simulink model "PIDdesign"  (R2019b)
settings: Solver=VariableStepAuto  StartTime=0.0  StopTime=5  RelTol=1e-3
values from neighbouring files (symbols this model uses):
  F2 = a*mass*g/(a+b)    (= 14.8072837402)    [main.m]
  g = 9.8    [EOM.m]    (also in main.m = 9.81)
  KDX = DesignVars(1,1).Value    [pidOptimization.m]
  KDY = DesignVars(2,1).Value    [pidOptimization.m]
  KIX = DesignVars(3,1).Value    [pidOptimization.m]
  KIY = DesignVars(4,1).Value    [pidOptimization.m]
  Kps = (Vmax-Vmin)/(Hmax-Hmin)    (= 1666.66666667)    [main.m]
  KPX = DesignVars(5,1).Value    [pidOptimization.m]
  KPY = DesignVars(6,1).Value    [pidOptimization.m]
  Ksv = 30    [main.m]
  nu = 1/h0    (= 20000)    [main.m]
  tau = 0.12    [main.m]
  Ts = 1/fs    (= 0.001)    [main.m]
  xeq = x(end,1)    [main.m]
  yeq = x(end,3)    [main.m]
undefined symbols (not defined in the file or in its folder): DiscIntNeverNeededParam
libraries: neural x106, simulink x4, checkpacklib x2
(part 3 of 3)

== system PIDdesign/NONLINEAR BEARING #2 WITHOUT UNBALANCE/BEARING 2 NL/B2NN/Layer 2/Delays 1 ==
  "p{2}" : Inport  PortDimensions=100
      mask Display: e = 0.06;c1 = [120 230 180]/255;c2 = ([120 230 180]+0)/(256+128);c3 = ([120 230 180]+128)/(256+128);patch([0 1 1 0],[0 0 1 1],c1);patch([0 1 1 1-e 1-e 0+e],[0 0 1 1-e 0+e 0+e],c2);patch([0 0 1 1-e 0+e 0+e],[0 1 1 1-e 1-e 0+e],c3);plot([0 1 1 0 0],[0 0 1 1 0]);
  mux : Mux  Inputs=1
      mask Display: e = 0.06;c1 = [120 150 230]/255;c2 = ([120 150 230]+0)/383;c3 = ([120 150 230]+128)/383;patch([0 1 1 0],[0 0 1 1],c1);patch([0 1 1 1-e 1-e 0+e],[0 0 1 1-e 0+e 0+e],c2);patch([0 0 1 1-e 0+e 0+e],[0 1 1 1-e 1-e 0+e],c3);plot([0 1 1 0 0],[0 0 1 1 0]);disp('Mux')
  "pd{2,1}" : Outport
      mask Display: e = 0.06;c1 = [120 230 180]/255;c2 = ([120 230 180]+0)/(256+128);c3 = ([120 230 180]+128)/(256+128);patch([0 1 1 0],[0 0 1 1],c1);patch([0 1 1 1-e 1-e 0+e],[0 0 1 1-e 0+e 0+e],c2);patch([0 0 1 1-e 0+e 0+e],[0 1 1 1-e 1-e 0+e],c3);plot([0 1 1 0 0],[0 0 1 1 0]);
  wires:
  "p{2}"/1 -> mux/1
  mux/1 -> "pd{2,1}"/1

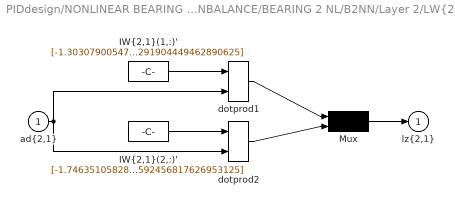
== system PIDdesign/NONLINEAR BEARING #2 WITHOUT UNBALANCE/BEARING 2 NL/B2NN/Layer 2/LW{2,1} ==
  "ad{2,1}" : Inport  PortDimensions=100
      mask Display: e = 0.06;c1 = [120 230 180]/255;c2 = ([120 230 180]+0)/(256+128);c3 = ([120 230 180]+128)/(256+128);patch([0 1 1 0],[0 0 1 1],c1);patch([0 1 1 1-e 1-e 0+e],[0 0 1 1-e 0+e 0+e],c2);patch([0 0 1 1-e 0+e 0+e],[0 1 1 1-e 1-e 0+e],c3);plot([0 1 1 0 0],[0 0 1 1 0]);
  "IW{2,1}(1,:)'" : Constant  Value=[-1.303079005476538210217540836310945451259613037109375;-0.8255005328617783799671769884298555552959442138671875;2.2416068989862178995053909602575004100799560546875;-0.55813390794967288055516974054626189172267913818359375;1.7083747820462615862879829364828765392303466796875;-5.33271180681637968490349521744064986705780029296875;1.93314459538238825331291081965900957584381103515625;-4.29747102149679438554130683769471943378448486328125;-1.835974747092809167270388570614159107208251953125;1.6115522585205634964466980818542651832103729248046875;-0.96088665944156925746710840030573308467864990234375;3.081953249444248310595639850362204015254974365234375;0.40542445031319385151391543331556022167205810546875;-2.371372573954384055383570739650167524814605712890625;0.2222251558369831292427676316947326995432376861572265625;-3.2786957332744872672947167302481830120086669921875;-0.65721019194913754546405471046455204486846923828125;4.5793081924106235902627304312773048877716064453125;3.396559076337279936552704384666867554187774658203125;-0.9506936842022923883632756769657135009765625;0.035530059029697712291717692778547643683850765228271484375;3.669635786509892749762684616143815219402313232421875;-1.0406028671959399733992768233292736113071441650390625;6.63327812826948548519112591748125851154327392578125;3.2833077579783580546290977508760988712310791015625;-1.003788449281528993850542974541895091533660888671875;1.5295131093832996516113098550704307854175567626953125;-0.292529913673766850390478566623642109334468841552734375;0.0103447720973679491152097398298792541027069091796875;-2.094937264749708649702597540454007685184478759765625;2.884830698716304819839706397033296525478363037109375;3.610348251303457711713917888118885457515716552734375;-0.65402756814988738387484090708312578499317169189453125;-0.2477855440938181164067799500116962008178234100341796875;1.469517455897823676735924891545437276363372802734375;-4.46176275310569980803165890392847359180450439453125;3.424182043452276946737811158527620136737823486328125;-5.45843716066573581002785431337542831897735595703125;-6.33904303768679344699421562836505472660064697265625;-4.5012635128892153346669147140346467494964599609375;3.136120918716373662249452536343596875667572021484375;1.571961496786693057714501264854334294795989990234375;-0.23371558494610022993498432697379030287265777587890625;-0.4635484960930360553987839011824689805507659912109375;3.23848369610364361648180420161224901676177978515625;2.509785332547937120040160152711905539035797119140625;2.960969019394504631037534636561758816242218017578125;3.81271075753365362714930597576312720775604248046875;0.87046392166746577867542100648279301822185516357421875;2.527528429159737743958658029441721737384796142578125;2.334886902139819309098811572766862809658050537109375;-2.2202064604060733898904800298623740673065185546875;-1.0971350826732237937477520972606725990772247314453125;5.3252075174508259891581474221311509609222412109375;1.9927529899432936399961135975900106132030487060546875;-1.7323109900493751656114227444049902260303497314453125;-5.2127254975364589739683651714585721492767333984375;3.613077625658748903703099131234921514987945556640625;-2.971965610222664366801836877129971981048583984375;1.9566041764405515124281009775586426258087158203125;0.8251166177697630832454933624831028282642364501953125;0.1193121441991285835992897546020685695111751556396484375;4.02380804450181717157875027623958885669708251953125;-1.0438645216073492161257263433071784675121307373046875;-0.477159922080958420753660220725578255951404571533203125;0.37484864586592514523744057441945187747478485107421875;-2.07618859433052183049994710017926990985870361328125;-3.19484410683969688449224122450686991214752197265625;0.5047112998937421934897429309785366058349609375;-0.181158393879384760349893213060568086802959442138671875;-3.09578760470798641790679539553821086883544921875;-1.4108370343958658299499120403197593986988067626953125;0.146634116610219356058308903811848722398281097412109375 ...(+1495 chars)]
      mask Display: e = 0.06;c1 = [120 150 230]/255;c2 = ([120 150 230]+0)/383;c3 = ([120 150 230]+128)/383;patch([0 1 1 0],[0 0 1 1],c1);patch([0 1 1 1-e 1-e 0+e],[0 0 1 1-e 0+e 0+e],c2);patch([0 0 1 1-e 0+e 0+e],[0 1 1 1-e 1-e 0+e],c3);plot([0 1 1 0 0],[0 0 1 1 0]);disp('weights');
  "IW{2,1}(2,:)'" : Constant  Value=[-1.7463510582880579224962502848939038813114166259765625;-0.3817553257546679734701911002048291265964508056640625;1.499441293389509155531413853168487548828125;0.59781227902492417580759820339153520762920379638671875;-1.572959088991725540296329199918545782566070556640625;-2.285896302660940904161179787479341030120849609375;0.1226153749453533225999279920870321802794933319091796875;0.48879224355486050601626857314840890467166900634765625;1.78087930741924349575810992973856627941131591796875;4.90264426696804722638489693053998053073883056640625;0.1678230741406869508391963563553872518241405487060546875;-5.99359077138990858912848125328309834003448486328125;-0.209639533671976519002555505721829831600189208984375;-0.8073258432726018174463433751952834427356719970703125;5.99096088644159152636348153464496135711669921875;1.47211352452196830853381470660679042339324951171875;4.13072350460404269512082464643754065036773681640625;1.3951298877763722572353799478150904178619384765625;0.267840609452006772617238539169193245470523834228515625;0.514410507555337570551046155742369592189788818359375;-8.597222996447595022573295864276587963104248046875;0.307005832961274205405999282447737641632556915283203125;1.0845127341180493818484364965115673840045928955078125;0.310722374666608847082471811518189497292041778564453125;1.1956344181233660162178011887590400874614715576171875;5.717061542137354734904874931089580059051513671875;-0.7872353439733881241835433684173040091991424560546875;-0.061544718284544497333143908690544776618480682373046875;-1.9906366295749784445234809027169831097126007080078125;-1.22258124482643903974121712963096797466278076171875;-1.515291638847875876905391123727895319461822509765625;2.7375042395839752629171925946138799190521240234375;-2.12826270114527460464159958064556121826171875;3.76220142421134529087112241541035473346710205078125;1.19249507911392971237773963366635143756866455078125;7.46450533719423159340067286393605172634124755859375;-1.57667617645866275921662236214615404605865478515625;0.13616106452400511539480021383496932685375213623046875;-0.03129722684529256948593456399976275861263275146484375;3.924354752442267280088117331615649163722991943359375;-6.7691416449166137425663691828958690166473388671875;1.455619350448965843014548227074556052684783935546875;0.1525039889476383636601752868955372832715511322021484375;3.81711921888099414701400746707804501056671142578125;-3.98679521713969808871524946880526840686798095703125;-4.23988796601051287638028952642343938350677490234375;1.1313598364804284823748048438574187457561492919921875;1.1338509882875762446730050214682705700397491455078125;-1.2873351419050964583590257461764849722385406494140625;-9.5250529974971502866765149519778788089752197265625;0.5386492857873672601698444850626401603221893310546875;-2.911503092256425784256634869961999356746673583984375;0.2278597588163693010709920372391934506595134735107421875;1.127643531196385051629249574034474790096282958984375;0.55780526308049738215544266495271585881710052490234375;5.93775110923110371885513814049772918224334716796875;0.16441798355035242007460283275577239692211151123046875;2.51670428144922642132996770669706165790557861328125;3.690456488905490051166680132155306637287139892578125;-6.58276106105876124274800531566143035888671875;-2.462614925171888291544064486515708267688751220703125;5.5107188605968957517688977532088756561279296875;1.381019801933926149928311133407987654209136962890625;4.75763931600114187148165001417510211467742919921875;-2.782763876646672684955774457193911075592041015625;3.306763994148273599904541697469539940357208251953125;-0.186539850676508522919760935110389254987239837646484375;3.029849029120091241651380187249742448329925537109375;0.2916556119648117118003938230685889720916748046875;1.9746781314328030187965623554191552102565765380859375;-1.8717633335384376014332019622088409960269927978515625;1.3419353608102879693575459896237589418888092041015625;-0.74501009632939396709616630687378346920013427734375 ...(+1460 chars)]
      mask Display: e = 0.06;c1 = [120 150 230]/255;c2 = ([120 150 230]+0)/383;c3 = ([120 150 230]+128)/383;patch([0 1 1 0],[0 0 1 1],c1);patch([0 1 1 1-e 1-e 0+e],[0 0 1 1-e 0+e 0+e],c2);patch([0 0 1 1-e 0+e 0+e],[0 1 1 1-e 1-e 0+e],c3);plot([0 1 1 0 0],[0 0 1 1 0]);disp('weights');
  Mux : Mux  Inputs=2
      mask Display: e = 0.06;c1 = [120 150 230]/255;c2 = ([120 150 230]+0)/383;c3 = ([120 150 230]+128)/383;patch([0 1 1 0],[0 0 1 1],c1);patch([0 1 1 1-e 1-e 0+e],[0 0 1 1-e 0+e 0+e],c2);patch([0 0 1 1-e 0+e 0+e],[0 1 1 1-e 1-e 0+e],c3);plot([0 1 1 0 0],[0 0 1 1 0]);disp('Mux');
  dotprod1 : neural/Weight Functions/dotprod
      settings: SourceProductName=Deep Learning Toolbox
  dotprod2 : neural/Weight Functions/dotprod
      settings: SourceProductName=Deep Learning Toolbox
  "lz{2,1}" : Outport
      mask Display: e = 0.06;c1 = [120 230 180]/255;c2 = ([120 230 180]+0)/(256+128);c3 = ([120 230 180]+128)/(256+128);patch([0 1 1 0],[0 0 1 1],c1);patch([0 1 1 1-e 1-e 0+e],[0 0 1 1-e 0+e 0+e],c2);patch([0 0 1 1-e 0+e 0+e],[0 1 1 1-e 1-e 0+e],c3);plot([0 1 1 0 0],[0 0 1 1 0]);
  wires:
  "IW{2,1}(1,:)'"/1 -> dotprod1/1
  "ad{2,1}"/1 -> dotprod1/2, dotprod2/2
  dotprod1/1 -> Mux/1
  "IW{2,1}(2,:)'"/1 -> dotprod2/1
  dotprod2/1 -> Mux/2
  Mux/1 -> "lz{2,1}"/1

== matlab function PIDdesign/REFERENCE SHAPING (cos) ==
  data: t input; t0 input; t1 input; Xc input; REFX output; Yc input; Xref input; Yref input; REFY output
function [REFX, REFY] = RefShaping(t,t0,t1,Xc,Yc,Xref,Yref)
Ax=(Xref-Xc)/2;
Ay=(Yref-Yc)/2;
w=pi/(t1-t0);

if t<t0
    REFX=Xc;
    REFY=Yc;
else if t>t1
        REFX=Xref;
        REFY=Yref;
    else
        REFX=Ax*cos(w*(t-t0)+pi)+(Xc+Ax);
        REFY=Ay*cos(w*(t-t0)+pi)+(Yc+Ay);
    end
end

== matlab function PIDdesign/STEP REFERENCE ==
  data: t input; t0 input; Xc input; REFX output; Yc input; Xref input; Yref input; REFY output
function [REFX, REFY] = StepReference(t,t0,Xc,Yc,Xref,Yref)
if t<t0
    REFX=Xc;
    REFY=Yc;
else
    REFX=Xref;
    REFY=Yref;
end
